simulink library "SCMS"  (R2017a)
settings: Solver=VariableStepAuto  StartTime=0.0  StopTime=10.0  RelTol=1e-3
values from neighbouring files (symbols this model uses):
  lt = 3    [examplesupplychainCIO.m]
  S = 2000    [examplesupplychainCIO.m]
undefined symbols (not defined in the file or in its folder): magnitude
undefined symbols (not defined in the file): norminv
settings Model: Creator=azken  LastModifiedBy=azken

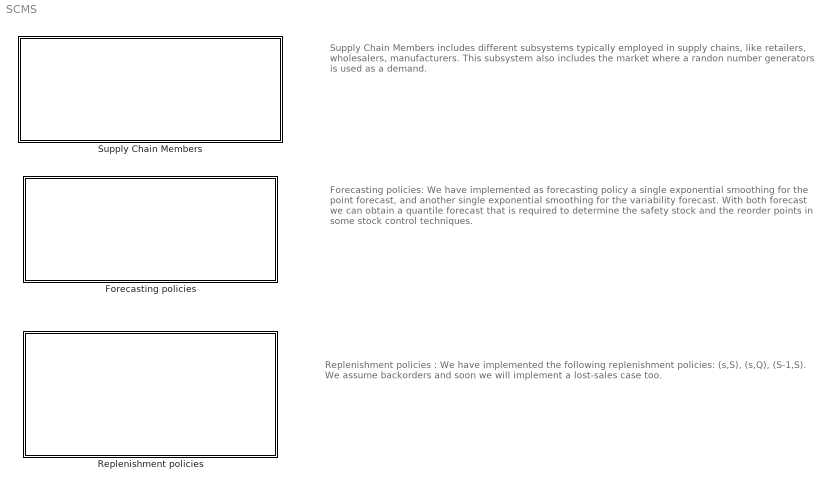
== system SCMS ==
  note: Forecasting policies: We have implemented as forecasting policy a single exponential smoothing for the point forecast, and another single exponential smoothing for the variability forecast. With both forecast we can obtain a quantile forecast that is required to determine the safety stock and the reorder points in some stock control techniques.
  note: Supply Chain Members includes different subsystems typically employed in supply chains, like retailers, wholesalers, manufacturers. This subsystem also includes the market where a randon number generators is used as a demand.
  note: Replenishment policies : We have implemented the following replenishment policies: (s,S), (s,Q), (S-1,S). We assume backorders and soon we will implement a lost-sales case too.
  Forecasting policies : Subsystem
  Replenishment policies : Subsystem
  Supply Chain Members : Subsystem

== system SCMS/Forecasting policies ==
  Forecast system with lead time (SES) : Subsystem  mask{alpha1=0.0, ini1=101.0713, alpha2=0.010, ini2=354.0398, k=2.3263, lt=4}
      mask prompts: alpha1 "SES constant (alpha1)"; alpha2 "SES constant (alpha2)"; k "safety factor (k)"; lt "lead time"
      mask help:
      | This block computes the lead time quantile forecast of the demand. Please, see the block help for more details about block parameters.
      | Usually the output of this block is fed to stock control blocks to determine the reorder point.
      mask Help:
      | Input: Demand
      | Output:
      |    Lead time quantile forecast.
      | Parameters:
      |    alpha1: exponential smoothing constant used to compute mean forecast.
      |    ini1: initial forecast used by exponential smoothing regarding mean forecast.
      |    alpha2: exponential smoothing constant used to compute variance forecast.
      |    ini2: initial forecast used by exponential smoothing regarding variance forecast.
      |    k: safety factor that depends on the cycle service level (quantile).
      |    lead time.

== system SCMS/Replenishment policies ==
  Stock control system (S-1,S) : Subsystem
  Stock control system (s,Q) : Subsystem  mask{Q=20}
  Stock control system (s,S) : Subsystem  mask{S=20}

== system SCMS/Supply Chain Members ==
  note: Market: It includes a random number generator as a demand generator and it receives the sales from the retailer
  note: Manufacturer : It receives its demand and provides the shipments. It is assumed that there is not any other company upwards, thus, it just has one input and one output. There is a delay implemented inside the Manufacturer block that simulates the elapsed time required to build/extract their products.
  note: Retailer/Wholesaler :
      | Inputs: Demand from Market (Retailer) and Shipments from Wholesarer (Manufacturer).
      | Outputs : Orders to Wholesaler (Manufacturer) and Sales to Market (Retailer)
      | Forecasting policy : Single exponential Smoothing.
      | Stock policy : (s,S)
      |
      | Retailer/Wholesaler promo may active a promotion that acts as an input for market promo. For this reason, this block has an extra output.
  note: Market Promo: It includes a random number generator as a demand generator and it receives the sales from the retailer. Additionally if input:promo in is active, an increase in sales is considered.
  Manufacturer : Subsystem
  Market : Subsystem
  Market Promo : Subsystem  AncestorBlock=SCMSv2016a/Supply Chain Members/Market
  Retailer : Subsystem
  Retailer promo : Subsystem  AncestorBlock=SCMSv2016a/Supply Chain Members/Retailer
  Wholesaler : Subsystem

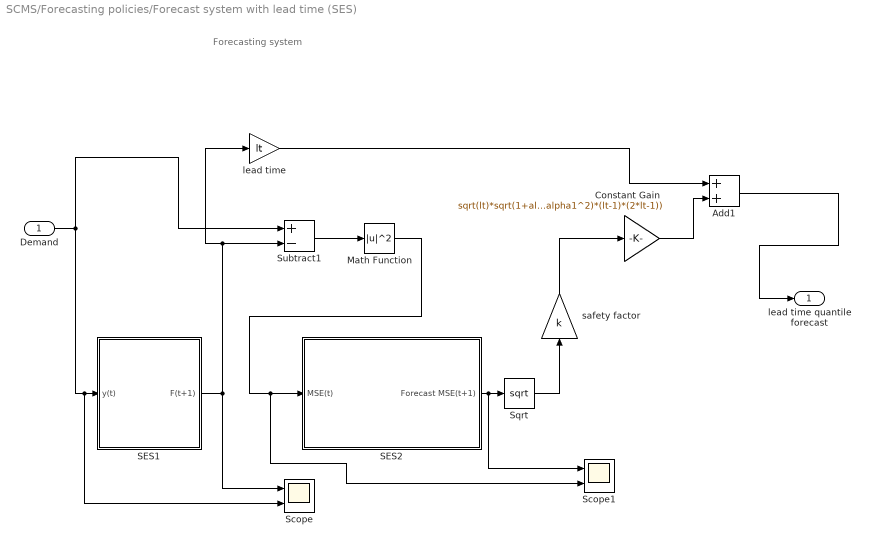
== system SCMS/Forecasting policies/Forecast system with lead time (SES) ==
  note: Forecasting system
  Demand : Inport
  Add1 : Sum
  Constant Gain : Gain  Gain=sqrt(lt)*sqrt(1+alpha1*(lt-1)+1/6*(alpha1^2)*(lt-1)*(2*lt-1))
  Math Function : Math  Operator=magnitude^2  SaturateOnIntegerOverflow=on
  SES1 : Subsystem
  SES2 : Subsystem
  Scope : Scope  NumInputPorts=2
  Scope1 : Scope  NumInputPorts=2
  Sqrt : Sqrt  SaturateOnIntegerOverflow=on
  Subtract1 : Sum  Inputs=+-
  lead time : Gain  Gain=lt
  safety factor : Gain  Gain=k
  lead time quantile forecast : Outport
  wires:
  Add1/1 -> lead time quantile forecast/1
  Constant Gain/1 -> Add1/2
  safety factor/1 -> Constant Gain/1
  lead time/1 -> Add1/1
  SES2/1(Forecast MSE(t+1)) -> Scope1/1, Sqrt/1
  Sqrt/1 -> safety factor/1
  Subtract1/1 -> Math Function/1
  Math Function/1 -> SES2/1(MSE(t)), Scope1/2
  SES1/1(F(t+1)) -> Subtract1/2, lead time/1, Scope/1
  Demand/1 -> Scope/2, SES1/1(y(t)), Subtract1/1

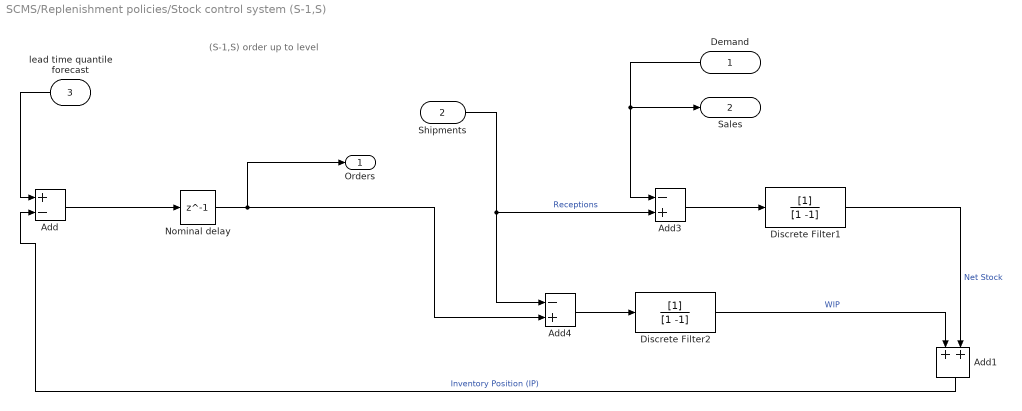
== system SCMS/Replenishment policies/Stock control system (S-1,S) ==
  note: (S-1,S) order up to level
  Demand : Inport
  Shipments : Inport  Port=2
  lead time quantile forecast : Inport  Port=3
  Add : Sum  Inputs=+-
  Add1 : Sum
  Add3 : Sum  Inputs=-+
  Add4 : Sum  Inputs=-+
  Discrete Filter1 : DiscreteFilter  Denominator=[1 -1]  SampleTime=1
  Discrete Filter2 : DiscreteFilter  Denominator=[1 -1]  SampleTime=1
  Nominal delay : Delay  DelayLength=1  InputProcessing=Inherited
  Orders : Outport
  Sales : Outport  Port=2
  wires:
  Discrete Filter2/1 -> Add1/1  "WIP"
  Shipments/1 -> Add3/2, Add4/1  "Receptions"
  Add1/1 -> Add/2  "Inventory Position (IP)"
  Discrete Filter1/1 -> Add1/2  "Net Stock"
  Nominal delay/1 -> Add4/2, Orders/1
  Add3/1 -> Discrete Filter1/1
  Demand/1 -> Add3/1, Sales/1
  Add4/1 -> Discrete Filter2/1
  lead time quantile forecast/1 -> Add/1
  Add/1 -> Nominal delay/1

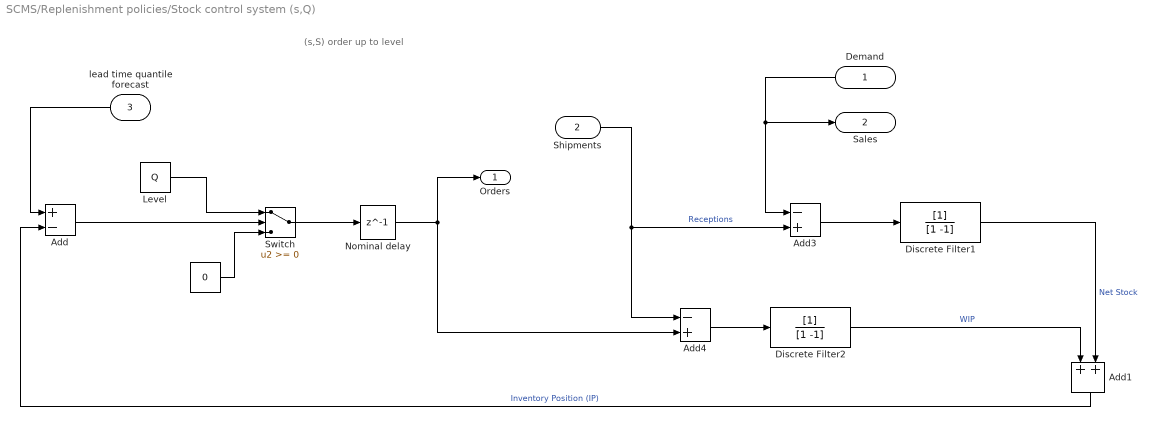
== system SCMS/Replenishment policies/Stock control system (s,Q) ==
  note: (s,S) order up to level
  Demand : Inport
  Shipments : Inport  Port=2
  lead time quantile forecast : Inport  Port=3
  " " : Constant  Value=0
  Add : Sum  Inputs=+-
  Add1 : Sum
  Add3 : Sum  Inputs=-+
  Add4 : Sum  Inputs=-+
  Discrete Filter1 : DiscreteFilter  Denominator=[1 -1]  SampleTime=1
  Discrete Filter2 : DiscreteFilter  Denominator=[1 -1]  SampleTime=1
  Level : Constant  Value=Q
  Nominal delay : Delay  DelayLength=1  InputProcessing=Inherited
  Switch : Switch
  Orders : Outport
  Sales : Outport  Port=2
  wires:
  Switch/1 -> Nominal delay/1
  Discrete Filter2/1 -> Add1/1  "WIP"
  Shipments/1 -> Add3/2, Add4/1  "Receptions"
  Level/1 -> Switch/1
  Add1/1 -> Add/2  "Inventory Position (IP)"
  Discrete Filter1/1 -> Add1/2  "Net Stock"
  Nominal delay/1 -> Add4/2, Orders/1
  Add/1 -> Switch/2
  Add3/1 -> Discrete Filter1/1
  Demand/1 -> Add3/1, Sales/1
  Add4/1 -> Discrete Filter2/1
  " "/1 -> Switch/3
  lead time quantile forecast/1 -> Add/1

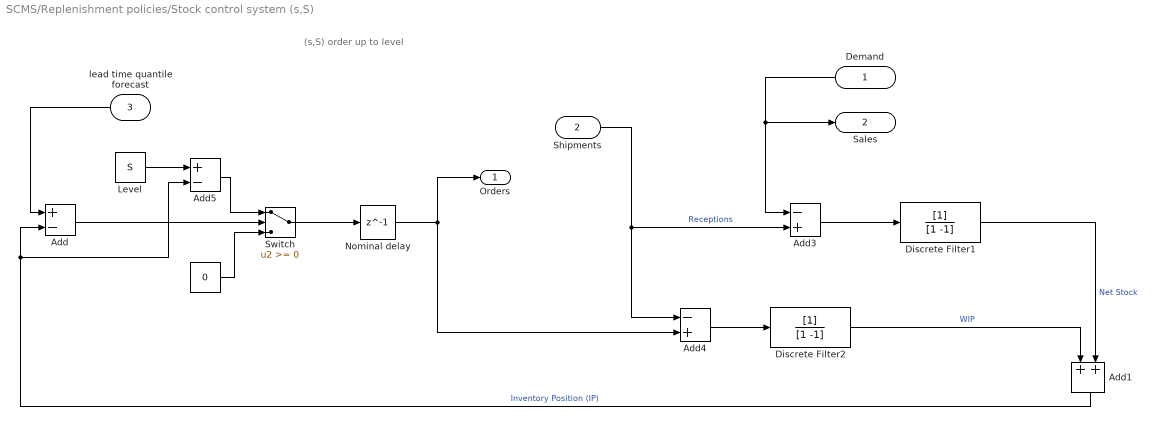
== system SCMS/Replenishment policies/Stock control system (s,S) ==
  note: (s,S) order up to level
  Demand : Inport
  Shipments : Inport  Port=2
  lead time quantile forecast : Inport  Port=3
  " " : Constant  Value=0
  Add : Sum  Inputs=+-
  Add1 : Sum
  Add3 : Sum  Inputs=-+
  Add4 : Sum  Inputs=-+
  Add5 : Sum  Inputs=+-
  Discrete Filter1 : DiscreteFilter  Denominator=[1 -1]  SampleTime=1
  Discrete Filter2 : DiscreteFilter  Denominator=[1 -1]  SampleTime=1
  Level : Constant  Value=S
  Nominal delay : Delay  DelayLength=1  InputProcessing=Inherited
  Switch : Switch
  Orders : Outport
  Sales : Outport  Port=2
  wires:
  Switch/1 -> Nominal delay/1
  Discrete Filter2/1 -> Add1/1  "WIP"
  Shipments/1 -> Add3/2, Add4/1  "Receptions"
  Add5/1 -> Switch/1
  Add1/1 -> Add/2, Add5/2  "Inventory Position (IP)"
  Discrete Filter1/1 -> Add1/2  "Net Stock"
  Nominal delay/1 -> Add4/2, Orders/1
  Add/1 -> Switch/2
  Level/1 -> Add5/1
  Add3/1 -> Discrete Filter1/1
  Demand/1 -> Add3/1, Sales/1
  Add4/1 -> Discrete Filter2/1
  " "/1 -> Switch/3
  lead time quantile forecast/1 -> Add/1

== system SCMS/Supply Chain Members/Manufacturer ==
  note: Manufacturer
  Demand : Inport
  Forecast system with lead time (SES) : Subsystem  mask{alpha1=0.1, ini1=101.0713, alpha2=0.01, ini2=354.0398, k=2.3263, lt=4}
      mask prompts: alpha1 "SES constant parameter (alpha1)"; ini1 "initialization SES for mean demand"; alpha2 "SES constant parameter (alpha2)"; ini2 "initialization SES for MSE"; k "Safety factor (k)"; lt "lead time"
      mask help: This block computes the lead time quantile forecast of the demand.
      mask Help:
      | Input: Demand
      | Output:
      |    Lead time quantile forecast.
      | Parameters:
      |    alpha1: exponential smoothing constant used to compute mean forecast.
      |    ini1: initial forecast used by exponential smoothing regarding mean forecast.
      |    alpha2: exponential smoothing constant used to compute variance forecast.
      |    ini2: initial forecast used by exponential smoothing regarding variance forecast.
      |    k: safety factor that depends on the cycle service level (quantile).
  Stock control system (s,S) : Subsystem  mask{S=15, Tp=2}
  Shipments : Outport
  wires:
  Stock control system (s,S)/1(Shipments) -> Shipments/1
  Forecast system with lead time (SES)/1(lead time quantile forecast) -> Stock control system (s,S)/2(lead time quantile forecast)
  Demand/1 -> Stock control system (s,S)/1(Demand), Forecast system with lead time (SES)/1(Demand)

== system SCMS/Supply Chain Members/Market ==
  Sales : Inport
  Random Number : RandomNumber  Mean=100  Variance=20  SampleTime=1
  Terminator2 : Terminator
  Demand : Outport
  wires:
  Random Number/1 -> Demand/1
  Sales/1 -> Terminator2/1

== system SCMS/Supply Chain Members/Market Promo ==
  note: This block containes the percentage increase of the promotion. By default is 20%
  Sales : Inport
  promo in : Inport  Port=2
  Base demand : RandomNumber  Mean=100  Variance=20  SampleTime=1
  If : If
  If Action Subsystem1 : Subsystem  TreatAsAtomicUnit=on
  Switch : Switch  Criteria=u2 > Threshold
  Terminator2 : Terminator
  demand increase : Subsystem  TreatAsAtomicUnit=on
  Demand : Outport
  wires:
  Sales/1 -> Terminator2/1
  promo in/1 -> Switch/2, If/1
  If/1 -> demand increase/Action
  If/2 -> If Action Subsystem1/Action
  Base demand/1 -> If Action Subsystem1/1(In1), demand increase/1(In2)
  Switch/1 -> Demand/1
  demand increase/1(Out1) -> Switch/1
  If Action Subsystem1/1(Out1) -> Switch/3

== system SCMS/Supply Chain Members/Retailer ==
  note: Retailer
  Demand : Inport
  Shipments : Inport  Port=2
  Forecast system with lead time (SES) : Subsystem  mask{alpha1=0.1, ini1=101.0713, alpha2=0.1, ini2=354.0398, k=2.3263, lt=4}
      mask prompts: lt "lead time"
      mask help: This block computes the mean and quantile forecast of the demand. The forecasting horizon is set to 1.
      mask Help:
      | Input: Demand
      | Output:
      |    Mean forecast.
      |    Quantile forecast.
      | Parameters:
      |    alpha1: exponential smoothing constant used to compute mean forecast.
      |    ini1: initial forecast used by exponential smoothing regarding mean forecast.
      |    alpha2: exponential smoothing constant used to compute variance forecast.
      |    ini2: initial forecast used by exponential smoothing regarding variance forecast.
      |    k: safety factor that depends on the cycle service level (quantile).
  Stock control system (s,S) : Subsystem  mask{S=20}
  Orders : Outport
  Sales : Outport  Port=2
  wires:
  Shipments/1 -> Stock control system (s,S)/2(Shipments)
  Stock control system (s,S)/1(Orders) -> Orders/1
  Stock control system (s,S)/2(Sales) -> Sales/1
  Forecast system with lead time (SES)/1(lead time quantile forecast) -> Stock control system (s,S)/3(lead time quantile forecast)
  Demand/1 -> Stock control system (s,S)/1(Demand), Forecast system with lead time (SES)/1(Demand)

== system SCMS/Supply Chain Members/Retailer promo ==
  note: This block is a dummy variable with ones for the periods where there is a promotion
  note: Retailer
  Demand : Inport
  Shipments : Inport  Port=2
  Forecast system with lead time (SES) : Subsystem  AncestorBlock=SCMSv2016a/Forecasting policies/Forecast system with lead time (SES)  mask{alpha1=0.1, ini1=100, alpha2=0.010, ini2=15, k=norminv(0.95,0,1), lt=3}
      mask prompts: alpha1 "SES constant (alpha1)"; alpha2 "SES constant (alpha2)"; k "safety factor (k)"; lt "lead time"
      mask help:
      | This block computes the lead time quantile forecast of the demand. Please, see the block help for more details about block parameters.
      | Usually the output of this block is fed to stock control blocks to determine the reorder point.
      mask Help:
      | Input: Demand
      | Output:
      |    Lead time quantile forecast.
      | Parameters:
      |    alpha1: exponential smoothing constant used to compute mean forecast.
      |    ini1: initial forecast used by exponential smoothing regarding mean forecast.
      |    alpha2: exponential smoothing constant used to compute variance forecast.
      |    ini2: initial forecast used by exponential smoothing regarding variance forecast.
      |    k: safety factor that depends on the cycle service level (quantile).
      |    lead time.
  From Workspace : FromWorkspace  VariableName=dummypromo  SampleTime=1
  Stock control system (s,S) : Subsystem  mask{S=1000}
  Orders : Outport
  Sales : Outport  Port=2
  promo active : Outport  Port=3
  wires:
  Demand/1 -> Stock control system (s,S)/1(Demand), Forecast system with lead time (SES)/1(Demand)
  Forecast system with lead time (SES)/1(lead time quantile forecast) -> Stock control system (s,S)/3(lead time quantile forecast)
  Stock control system (s,S)/2(Sales) -> Sales/1
  Stock control system (s,S)/1(Orders) -> Orders/1
  Shipments/1 -> Stock control system (s,S)/2(Shipments)
  From Workspace/1 -> promo active/1

== system SCMS/Supply Chain Members/Wholesaler ==
  note: Retailer
  Demand : Inport
  Shipments manufacturer : Inport  Port=2
  Forecast system with lead time (SES) : Subsystem  mask{alpha1=0.1, ini1=101.0713, alpha2=0.01, ini2=354.0398, k=2.3263, lt=lt}
      mask prompts: lt "lead time"
      mask help: This block computes the mean and quantile forecast of the demand. The forecasting horizon is set to 1.
      mask Help:
      | Input: Demand
      | Output:
      |    Mean forecast.
      |    Quantile forecast.
      | Parameters:
      |    alpha1: exponential smoothing constant used to compute mean forecast.
      |    ini1: initial forecast used by exponential smoothing regarding mean forecast.
      |    alpha2: exponential smoothing constant used to compute variance forecast.
      |    ini2: initial forecast used by exponential smoothing regarding variance forecast.
      |    k: safety factor that depends on the cycle service level (quantile).
  Stock control system (s,S) : Subsystem
  Orders : Outport
  Shipments wholesaler : Outport  Port=2
  wires:
  Shipments manufacturer/1 -> Stock control system (s,S)/2(Shipments)
  Stock control system (s,S)/1(Orders) -> Orders/1
  Stock control system (s,S)/2(Sales) -> Shipments wholesaler/1
  Forecast system with lead time (SES)/1(lead time quantile forecast) -> Stock control system (s,S)/3(lead time quantile forecast)
  Demand/1 -> Stock control system (s,S)/1(Demand), Forecast system with lead time (SES)/1(Demand)

== system SCMS/Forecasting policies/Forecast system with lead time (SES)/SES1 ==
  note: Demand
  note: Forecast
  note: Simple Exponential Smoothing
  y(t) : Inport
  Add : Sum
  Delay : Delay  DelayLength=1  InitialCondition=ini1
  Gain : Gain  Gain=(1-alpha1)
  Gain1 : Gain  Gain=alpha1
  F(t+1) : Outport
  wires:
  Add/1 -> Delay/1, F(t+1)/1
  y(t)/1 -> Gain1/1
  Gain1/1 -> Add/2
  Delay/1 -> Gain/1
  Gain/1 -> Add/1

== system SCMS/Forecasting policies/Forecast system with lead time (SES)/SES2 ==
  MSE(t) : Inport
  Add : Sum
  Delay : Delay  DelayLength=1  InitialCondition=ini2
  Gain : Gain  Gain=(1-alpha2)
  Gain1 : Gain  Gain=alpha2
  Forecast MSE(t+1) : Outport
  wires:
  Add/1 -> Delay/1, Forecast MSE(t+1)/1
  MSE(t)/1 -> Gain1/1
  Gain1/1 -> Add/2
  Delay/1 -> Gain/1
  Gain/1 -> Add/1

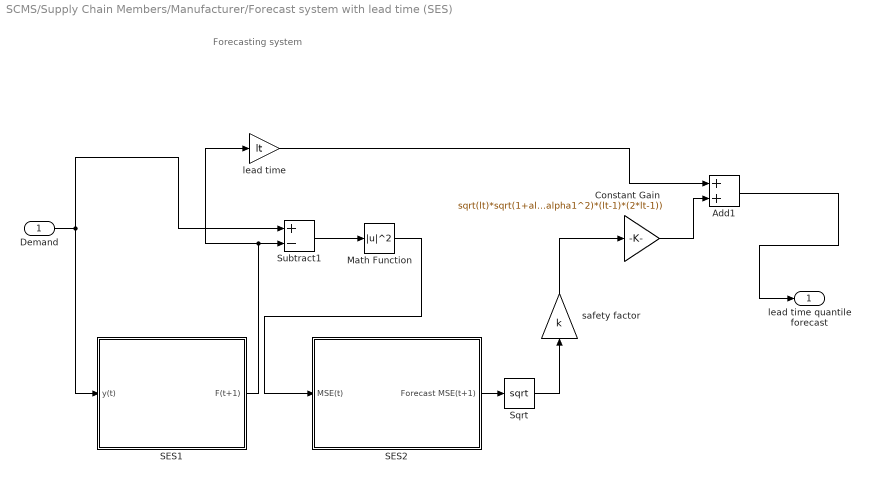
== system SCMS/Supply Chain Members/Manufacturer/Forecast system with lead time (SES) ==
  note: Forecasting system
  Demand : Inport
  Add1 : Sum
  Constant Gain : Gain  Gain=sqrt(lt)*sqrt(1+alpha1*(lt-1)+1/6*(alpha1^2)*(lt-1)*(2*lt-1))
  Math Function : Math  Operator=magnitude^2  SaturateOnIntegerOverflow=on
  SES1 : Subsystem
  SES2 : Subsystem
  Sqrt : Sqrt  SaturateOnIntegerOverflow=on
  Subtract1 : Sum  Inputs=+-
  lead time : Gain  Gain=lt
  safety factor : Gain  Gain=k
  lead time quantile forecast : Outport
  wires:
  Add1/1 -> lead time quantile forecast/1
  Constant Gain/1 -> Add1/2
  safety factor/1 -> Constant Gain/1
  lead time/1 -> Add1/1
  SES2/1(Forecast MSE(t+1)) -> Sqrt/1
  Sqrt/1 -> safety factor/1
  Subtract1/1 -> Math Function/1
  Math Function/1 -> SES2/1(MSE(t))
  SES1/1(F(t+1)) -> Subtract1/2, lead time/1
  Demand/1 -> SES1/1(y(t)), Subtract1/1

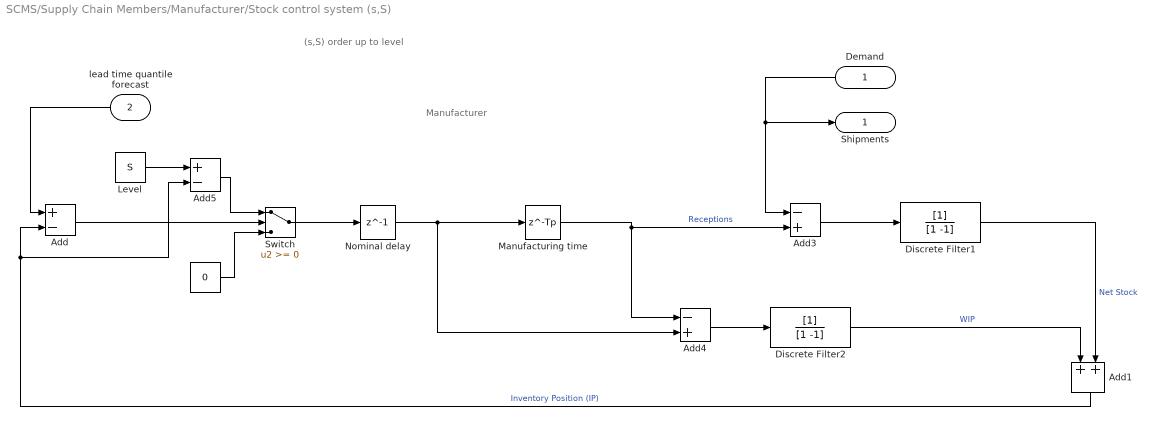
== system SCMS/Supply Chain Members/Manufacturer/Stock control system (s,S) ==
  note: Manufacturer
  note: (s,S) order up to level
  Demand : Inport
  lead time quantile forecast : Inport  Port=2
  " " : Constant  Value=0
  Add : Sum  Inputs=+-
  Add1 : Sum
  Add3 : Sum  Inputs=-+
  Add4 : Sum  Inputs=-+
  Add5 : Sum  Inputs=+-
  Discrete Filter1 : DiscreteFilter  Denominator=[1 -1]  SampleTime=1
  Discrete Filter2 : DiscreteFilter  Denominator=[1 -1]  SampleTime=1
  Level : Constant  Value=S
  Manufacturing time : Delay  DelayLength=Tp  InputProcessing=Inherited
  Nominal delay : Delay  DelayLength=1  InputProcessing=Inherited
  Switch : Switch
  Shipments : Outport
  wires:
  Switch/1 -> Nominal delay/1
  Discrete Filter2/1 -> Add1/1  "WIP"
  Manufacturing time/1 -> Add3/2, Add4/1  "Receptions"
  Add5/1 -> Switch/1
  Add1/1 -> Add/2, Add5/2  "Inventory Position (IP)"
  Discrete Filter1/1 -> Add1/2  "Net Stock"
  Nominal delay/1 -> Manufacturing time/1, Add4/2
  Add/1 -> Switch/2
  Level/1 -> Add5/1
  Add3/1 -> Discrete Filter1/1
  Demand/1 -> Add3/1, Shipments/1
  Add4/1 -> Discrete Filter2/1
  " "/1 -> Switch/3
  lead time quantile forecast/1 -> Add/1

== system SCMS/Supply Chain Members/Market Promo/If Action Subsystem1 ==
  In1 : Inport
  Action Port : ActionPort
  Out1 : Outport
  wires:
  In1/1 -> Out1/1

== system SCMS/Supply Chain Members/Market Promo/demand increase ==
  In2 : Inport
  Action Port : ActionPort
  Gain : Gain  Gain=1.2
  Out1 : Outport
  wires:
  In2/1 -> Gain/1
  Gain/1 -> Out1/1

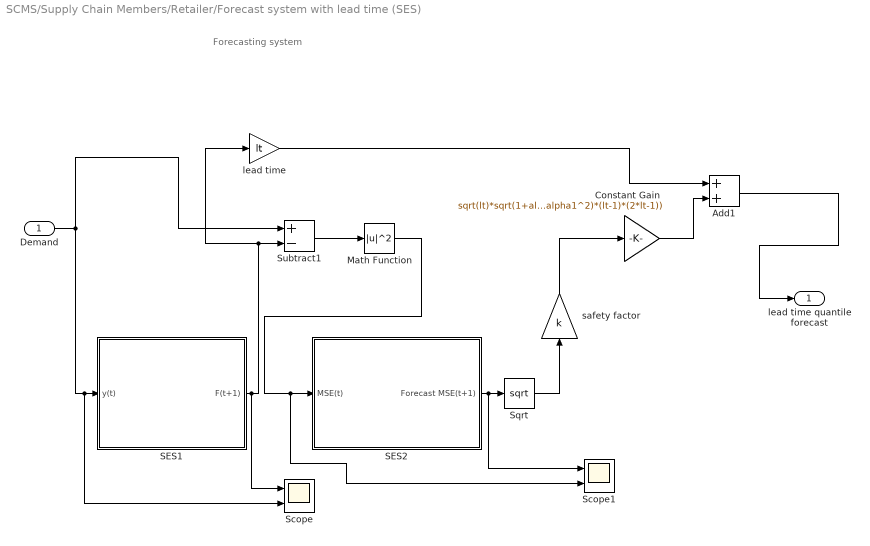
== system SCMS/Supply Chain Members/Retailer/Forecast system with lead time (SES) ==
  note: Forecasting system
  Demand : Inport
  Add1 : Sum
  Constant Gain : Gain  Gain=sqrt(lt)*sqrt(1+alpha1*(lt-1)+1/6*(alpha1^2)*(lt-1)*(2*lt-1))
  Math Function : Math  Operator=magnitude^2  SaturateOnIntegerOverflow=on
  SES1 : Subsystem
  SES2 : Subsystem
  Scope : Scope  NumInputPorts=2
  Scope1 : Scope  NumInputPorts=2
  Sqrt : Sqrt  SaturateOnIntegerOverflow=on
  Subtract1 : Sum  Inputs=+-
  lead time : Gain  Gain=lt
  safety factor : Gain  Gain=k
  lead time quantile forecast : Outport
  wires:
  Add1/1 -> lead time quantile forecast/1
  Constant Gain/1 -> Add1/2
  safety factor/1 -> Constant Gain/1
  lead time/1 -> Add1/1
  SES2/1(Forecast MSE(t+1)) -> Scope1/1, Sqrt/1
  Sqrt/1 -> safety factor/1
  Subtract1/1 -> Math Function/1
  Math Function/1 -> Scope1/2, SES2/1(MSE(t))
  SES1/1(F(t+1)) -> Scope/1, Subtract1/2, lead time/1
  Demand/1 -> Scope/2, SES1/1(y(t)), Subtract1/1

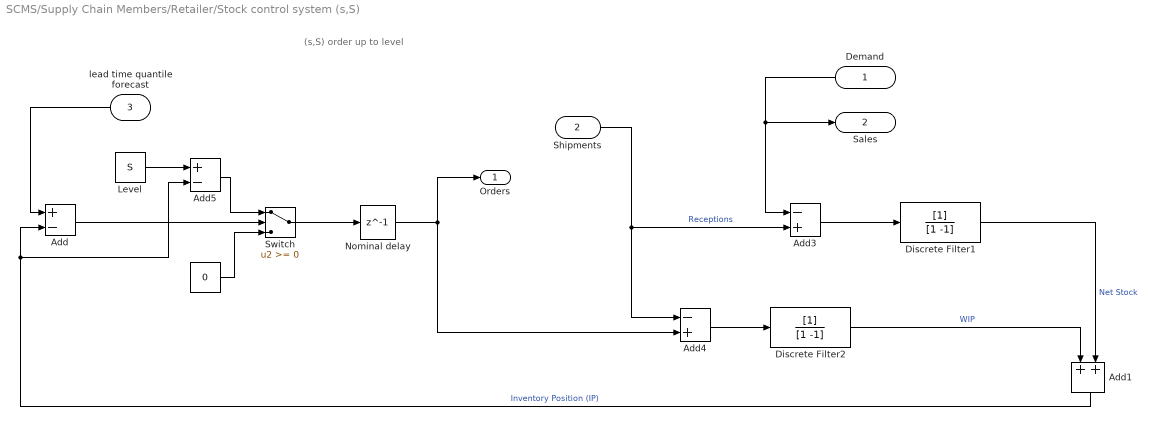
== system SCMS/Supply Chain Members/Retailer/Stock control system (s,S) ==
  note: (s,S) order up to level
  Demand : Inport
  Shipments : Inport  Port=2
  lead time quantile forecast : Inport  Port=3
  " " : Constant  Value=0
  Add : Sum  Inputs=+-
  Add1 : Sum
  Add3 : Sum  Inputs=-+
  Add4 : Sum  Inputs=-+
  Add5 : Sum  Inputs=+-
  Discrete Filter1 : DiscreteFilter  Denominator=[1 -1]  SampleTime=1
  Discrete Filter2 : DiscreteFilter  Denominator=[1 -1]  SampleTime=1
  Level : Constant  Value=S
  Nominal delay : Delay  DelayLength=1  InputProcessing=Inherited
  Switch : Switch
  Orders : Outport
  Sales : Outport  Port=2
  wires:
  Switch/1 -> Nominal delay/1
  Discrete Filter2/1 -> Add1/1  "WIP"
  Shipments/1 -> Add3/2, Add4/1  "Receptions"
  Add5/1 -> Switch/1
  Add1/1 -> Add/2, Add5/2  "Inventory Position (IP)"
  Discrete Filter1/1 -> Add1/2  "Net Stock"
  Nominal delay/1 -> Add4/2, Orders/1
  Add/1 -> Switch/2
  Level/1 -> Add5/1
  Add3/1 -> Discrete Filter1/1
  Demand/1 -> Add3/1, Sales/1
  Add4/1 -> Discrete Filter2/1
  " "/1 -> Switch/3
  lead time quantile forecast/1 -> Add/1

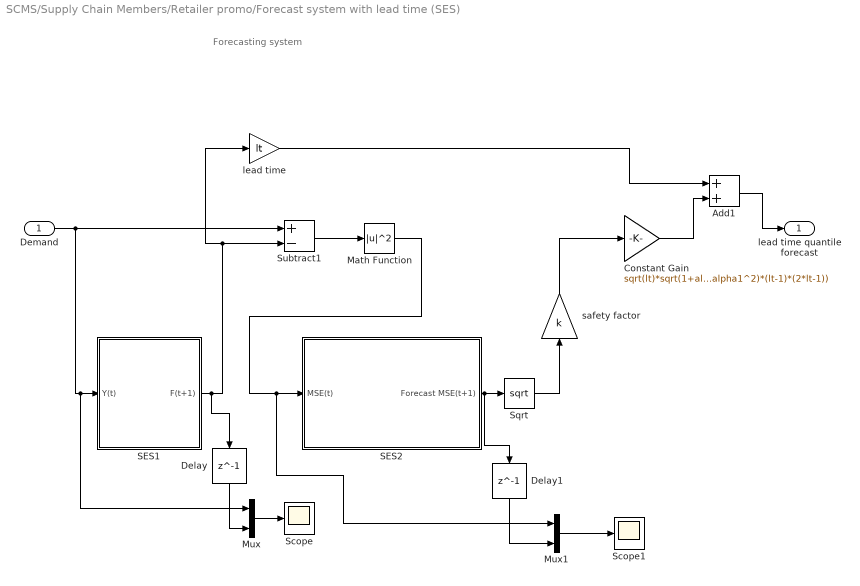
== system SCMS/Supply Chain Members/Retailer promo/Forecast system with lead time (SES) ==
  note: Forecasting system
  Demand : Inport
  Add1 : Sum
  Constant Gain : Gain  Gain=sqrt(lt)*sqrt(1+alpha1*(lt-1)+1/6*(alpha1^2)*(lt-1)*(2*lt-1))
  Delay : Delay  DelayLength=1  InitialCondition=ini1
  Delay1 : Delay  DelayLength=1  InitialCondition=ini2
  Math Function : Math  Operator=magnitude^2  SaturateOnIntegerOverflow=on
  Mux : Mux  Inputs=2
  Mux1 : Mux  Inputs=2
  SES1 : Subsystem
  SES2 : Subsystem
  Scope : Scope
  Scope1 : Scope
  Sqrt : Sqrt  SaturateOnIntegerOverflow=on
  Subtract1 : Sum  Inputs=+-
  lead time : Gain  Gain=lt
  safety factor : Gain  Gain=k
  lead time quantile forecast : Outport
  wires:
  Add1/1 -> lead time quantile forecast/1
  Constant Gain/1 -> Add1/2
  safety factor/1 -> Constant Gain/1
  lead time/1 -> Add1/1
  SES2/1(Forecast MSE(t+1)) -> Delay1/1, Sqrt/1
  Sqrt/1 -> safety factor/1
  Subtract1/1 -> Math Function/1
  Math Function/1 -> Mux1/1, SES2/1(MSE(t))
  SES1/1(F(t+1)) -> Delay/1, Subtract1/2, lead time/1
  Demand/1 -> Mux/1, SES1/1(Y(t)), Subtract1/1
  Mux1/1 -> Scope1/1
  Mux/1 -> Scope/1
  Delay/1 -> Mux/2
  Delay1/1 -> Mux1/2

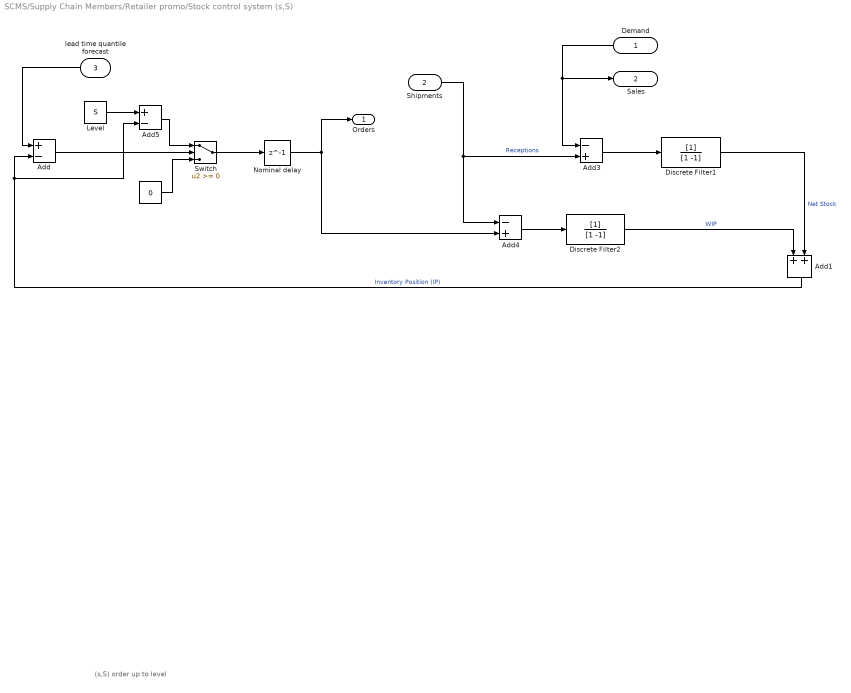
== system SCMS/Supply Chain Members/Retailer promo/Stock control system (s,S) ==
  note: (s,S) order up to level
  Demand : Inport
  Shipments : Inport  Port=2
  lead time quantile forecast : Inport  Port=3
  " " : Constant  Value=0
  Add : Sum  Inputs=+-
  Add1 : Sum
  Add3 : Sum  Inputs=-+
  Add4 : Sum  Inputs=-+
  Add5 : Sum  Inputs=+-
  Discrete Filter1 : DiscreteFilter  Denominator=[1 -1]  SampleTime=1
  Discrete Filter2 : DiscreteFilter  Denominator=[1 -1]  SampleTime=1
  Level : Constant  Value=S
  Nominal delay : Delay  DelayLength=1  InputProcessing=Inherited
  Switch : Switch
  Orders : Outport
  Sales : Outport  Port=2
  wires:
  lead time quantile forecast/1 -> Add/1
  " "/1 -> Switch/3
  Add4/1 -> Discrete Filter2/1
  Demand/1 -> Sales/1, Add3/1
  Add3/1 -> Discrete Filter1/1
  Level/1 -> Add5/1
  Add/1 -> Switch/2
  Nominal delay/1 -> Orders/1, Add4/2
  Discrete Filter1/1 -> Add1/2  "Net Stock"
  Add1/1 -> Add5/2, Add/2  "Inventory Position (IP)"
  Add5/1 -> Switch/1
  Shipments/1 -> Add4/1, Add3/2  "Receptions"
  Discrete Filter2/1 -> Add1/1  "WIP"
  Switch/1 -> Nominal delay/1

== system SCMS/Supply Chain Members/Wholesaler/Forecast system with lead time (SES) ==
  note: Forecasting system
  Demand : Inport
  Add1 : Sum
  Constant Gain : Gain  Gain=sqrt(lt)*sqrt(1+alpha1*(lt-1)+1/6*(alpha1^2)*(lt-1)*(2*lt-1))
  Math Function : Math  Operator=magnitude^2  SaturateOnIntegerOverflow=on
  SES1 : Subsystem
  SES2 : Subsystem
  Sqrt : Sqrt  SaturateOnIntegerOverflow=on
  Subtract1 : Sum  Inputs=+-
  lead time : Gain  Gain=lt
  safety factor : Gain  Gain=k
  lead time quantile forecast : Outport
  wires:
  Add1/1 -> lead time quantile forecast/1
  Constant Gain/1 -> Add1/2
  safety factor/1 -> Constant Gain/1
  lead time/1 -> Add1/1
  SES2/1(Forecast MSE(t+1)) -> Sqrt/1
  Sqrt/1 -> safety factor/1
  Subtract1/1 -> Math Function/1
  Math Function/1 -> SES2/1(MSE(t))
  SES1/1(F(t+1)) -> Subtract1/2, lead time/1
  Demand/1 -> SES1/1(y(t)), Subtract1/1

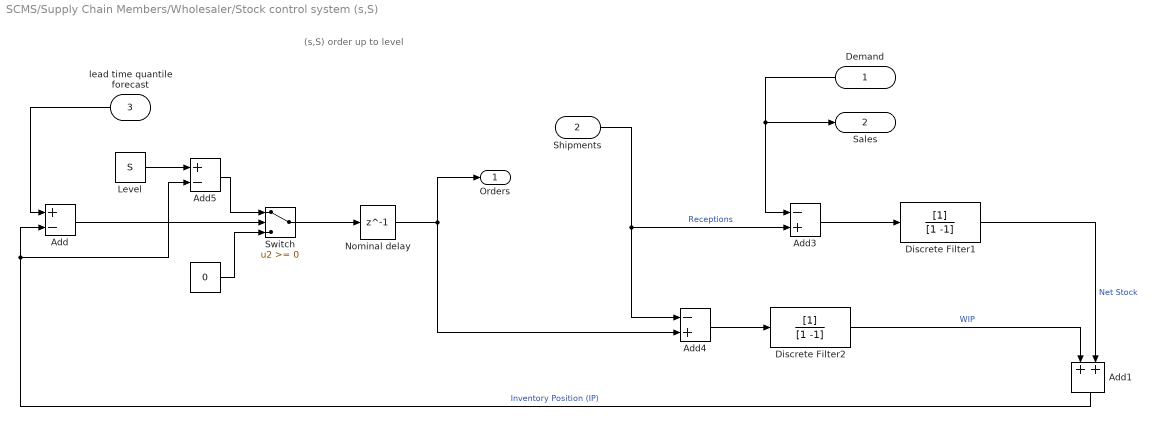
== system SCMS/Supply Chain Members/Wholesaler/Stock control system (s,S) ==
  note: (s,S) order up to level
  Demand : Inport
  Shipments : Inport  Port=2
  lead time quantile forecast : Inport  Port=3
  " " : Constant  Value=0
  Add : Sum  Inputs=+-
  Add1 : Sum
  Add3 : Sum  Inputs=-+
  Add4 : Sum  Inputs=-+
  Add5 : Sum  Inputs=+-
  Discrete Filter1 : DiscreteFilter  Denominator=[1 -1]  SampleTime=1
  Discrete Filter2 : DiscreteFilter  Denominator=[1 -1]  SampleTime=1
  Level : Constant  Value=S
  Nominal delay : Delay  DelayLength=1  InputProcessing=Inherited
  Switch : Switch
  Orders : Outport
  Sales : Outport  Port=2
  wires:
  Switch/1 -> Nominal delay/1
  Discrete Filter2/1 -> Add1/1  "WIP"
  Shipments/1 -> Add3/2, Add4/1  "Receptions"
  Add5/1 -> Switch/1
  Add1/1 -> Add/2, Add5/2  "Inventory Position (IP)"
  Discrete Filter1/1 -> Add1/2  "Net Stock"
  Nominal delay/1 -> Add4/2, Orders/1
  Add/1 -> Switch/2
  Level/1 -> Add5/1
  Add3/1 -> Discrete Filter1/1
  Demand/1 -> Add3/1, Sales/1
  Add4/1 -> Discrete Filter2/1
  " "/1 -> Switch/3
  lead time quantile forecast/1 -> Add/1

== system SCMS/Supply Chain Members/Manufacturer/Forecast system with lead time (SES)/SES1 ==
  note: Demand
  note: Forecast
  note: Simple Exponential Smoothing
  y(t) : Inport
  Add : Sum
  Delay : Delay  DelayLength=1  InitialCondition=ini1
  Gain : Gain  Gain=(1-alpha1)
  Gain1 : Gain  Gain=alpha1
  F(t+1) : Outport
  wires:
  Add/1 -> Delay/1, F(t+1)/1
  y(t)/1 -> Gain1/1
  Gain1/1 -> Add/2
  Delay/1 -> Gain/1
  Gain/1 -> Add/1

== system SCMS/Supply Chain Members/Manufacturer/Forecast system with lead time (SES)/SES2 ==
  MSE(t) : Inport
  Add : Sum
  Delay : Delay  DelayLength=1  InitialCondition=ini2
  Gain : Gain  Gain=(1-alpha2)
  Gain1 : Gain  Gain=alpha2
  Forecast MSE(t+1) : Outport
  wires:
  Add/1 -> Delay/1, Forecast MSE(t+1)/1
  MSE(t)/1 -> Gain1/1
  Gain1/1 -> Add/2
  Delay/1 -> Gain/1
  Gain/1 -> Add/1

== system SCMS/Supply Chain Members/Retailer/Forecast system with lead time (SES)/SES1 ==
  note: Demand
  note: Forecast
  note: Simple Exponential Smoothing
  y(t) : Inport
  Add : Sum
  Delay : Delay  DelayLength=1  InitialCondition=ini1
  Gain : Gain  Gain=(1-alpha1)
  Gain1 : Gain  Gain=alpha1
  F(t+1) : Outport
  wires:
  Add/1 -> Delay/1, F(t+1)/1
  y(t)/1 -> Gain1/1
  Gain1/1 -> Add/2
  Delay/1 -> Gain/1
  Gain/1 -> Add/1

== system SCMS/Supply Chain Members/Retailer/Forecast system with lead time (SES)/SES2 ==
  MSE(t) : Inport
  Add : Sum
  Delay : Delay  DelayLength=1  InitialCondition=ini2
  Gain : Gain  Gain=(1-alpha2)
  Gain1 : Gain  Gain=alpha2
  Forecast MSE(t+1) : Outport
  wires:
  Add/1 -> Delay/1, Forecast MSE(t+1)/1
  MSE(t)/1 -> Gain1/1
  Gain1/1 -> Add/2
  Delay/1 -> Gain/1
  Gain/1 -> Add/1

== system SCMS/Supply Chain Members/Retailer promo/Forecast system with lead time (SES)/SES1 ==
  note: Demand
  note: Forecast
  note: Simple Exponential Smoothing
  Y(t) : Inport
  Add : Sum
  Delay : Delay  DelayLength=1  InitialCondition=ini1
  Gain : Gain  Gain=(1-alpha1)
  Gain1 : Gain  Gain=alpha1
  F(t+1) : Outport
  wires:
  Add/1 -> Delay/1, F(t+1)/1
  Y(t)/1 -> Gain1/1
  Gain1/1 -> Add/2
  Delay/1 -> Gain/1
  Gain/1 -> Add/1

== system SCMS/Supply Chain Members/Retailer promo/Forecast system with lead time (SES)/SES2 ==
  MSE(t) : Inport
  Add : Sum
  Delay : Delay  DelayLength=1  InitialCondition=ini2
  Gain : Gain  Gain=(1-alpha2)
  Gain1 : Gain  Gain=alpha2
  Forecast MSE(t+1) : Outport
  wires:
  Add/1 -> Delay/1, Forecast MSE(t+1)/1
  MSE(t)/1 -> Gain1/1
  Gain1/1 -> Add/2
  Delay/1 -> Gain/1
  Gain/1 -> Add/1

== system SCMS/Supply Chain Members/Wholesaler/Forecast system with lead time (SES)/SES1 ==
  note: Demand
  note: Forecast
  note: Simple Exponential Smoothing
  y(t) : Inport
  Add : Sum
  Delay : Delay  DelayLength=1  InitialCondition=ini1
  Gain : Gain  Gain=(1-alpha1)
  Gain1 : Gain  Gain=alpha1
  F(t+1) : Outport
  wires:
  Add/1 -> Delay/1, F(t+1)/1
  y(t)/1 -> Gain1/1
  Gain1/1 -> Add/2
  Delay/1 -> Gain/1
  Gain/1 -> Add/1

== system SCMS/Supply Chain Members/Wholesaler/Forecast system with lead time (SES)/SES2 ==
  MSE(t) : Inport
  Add : Sum
  Delay : Delay  DelayLength=1  InitialCondition=ini2
  Gain : Gain  Gain=(1-alpha2)
  Gain1 : Gain  Gain=alpha2
  Forecast MSE(t+1) : Outport
  wires:
  Add/1 -> Delay/1, Forecast MSE(t+1)/1
  MSE(t)/1 -> Gain1/1
  Gain1/1 -> Add/2
  Delay/1 -> Gain/1
  Gain/1 -> Add/1
